simulink model "SafetyModule_Test"  (R2025b)
settings: Solver=VariableStepAuto  StartTime=0.0  StopTime=10.0  FixedStep=0.01  MaxStep=0.01  RelTol=1e-3
settings Model: Creator=mateu  LastModifiedBy=mateu

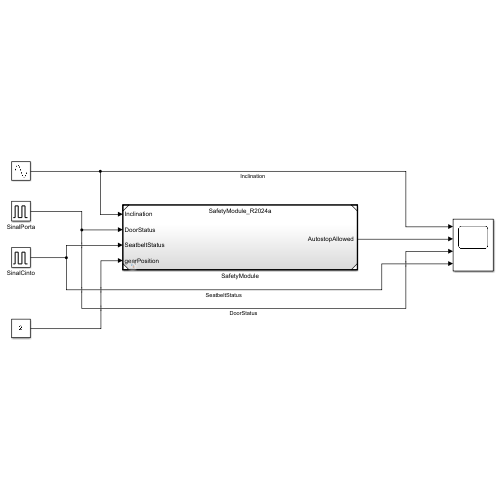
[thumbnail: Simulink's stored preview of the top-level diagram]
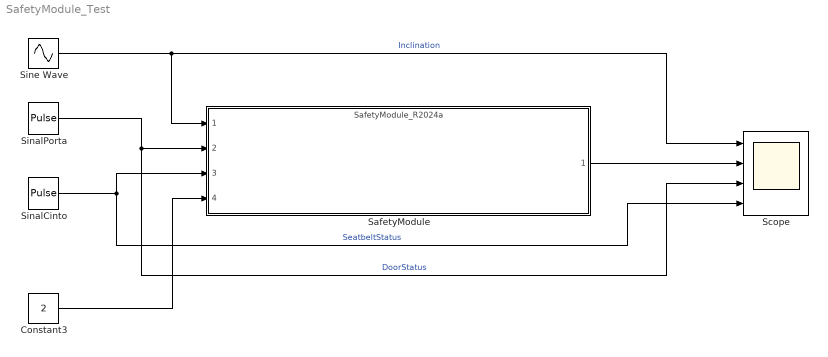
== system SafetyModule_Test ==
  Constant3 : Constant  Value=2
  SafetyModule : ModelReference  ModelNameDialog=SafetyModule_R2024a.slx  SimulationMode=Normal  ModelReferenceVersion=4.8
  Scope : Scope  NumInputPorts=4
      settings: ActiveDisplayString=4  ActiveDisplayYMinimum=-0.14932008082802595  ActiveDisplayYMaximum=1.0090678896298781
  SinalCinto : DiscretePulseGenerator  PulseType=Time based  PulseWidth=50
  SinalPorta : DiscretePulseGenerator  PulseType=Time based  Period=1  PulseWidth=50  PhaseDelay=0.5
  Sine Wave : Sin  Frequency=10  SampleTime=0
  wires:
  Sine Wave/1 -> Scope/1, SafetyModule/1  "Inclination"
  SinalPorta/1 -> SafetyModule/2, Scope/3  "DoorStatus"
  SafetyModule/1 -> Scope/2
  Constant3/1 -> SafetyModule/4
  SinalCinto/1 -> Scope/4, SafetyModule/3  "SeatbeltStatus"
